simulink model "StopwatchAndrea"  (R2018b)
settings: Solver=FixedStepAuto  StartTime=0.0  StopTime=Inf  FixedStep=0.1  RelTol=1e-3
libraries: simulink x1
settings Model: Creator=user  LastModifiedBy=Andrea Stevanato
settings DataIOCC: LimitDataPoints=on
settings OptimizationCC: DefaultParameterBehavior=Inlined  EnhancedBackFolding=on  PassReuseOutputArgsAs=Individual arguments  OptimizeBlockOrder=speed  DifferentSizesBufferReuse=on  OptimizationCustomize=off
settings DebuggingCC: ParameterTunabilityLossMsg=error  AllowSymbolicDim=off  SFUnexpectedBacktrackingDiag=warning  SFNoUnconditionalDefaultTransitionDiag=warning  SFExecutionAtInitializationDiag=none
settings ModelReferenceCC: PropagateSignalLabelsOutOfModel=off
settings SFSimCC: SimUseLocalCustomCode=off  MATLABDynamicMemAlloc=off
settings RTWCC: SystemTargetFile=ert.tlc  GenCodeOnly=on  TemplateMakefile=ert_default_tmf  GenerateReport=on  RTWUseLocalCustomCode=off  IncludeHyperlinkInReport=on  LaunchReport=on  GenerateTraceInfo=on  GenerateTraceReport=on  GenerateTraceReportSl=on  GenerateTraceReportSf=on  GenerateTraceReportEml=on
settings CodeAppCC: ForceParamTrailComments=on  IgnoreCustomStorageClasses=off  OperatorAnnotations=on  SimulinkDataObjDesc=on  SFDataObjDesc=on  InsertBlockDesc=on
settings ERTTargetCC: IncludeMdlTerminateFcn=off  SupportAbsoluteTime=off  MultiInstanceERTCode=on  CodeInterfacePackaging=Reusable function  PurelyIntegerCode=on  SupportNonFinite=off  SupportComplex=off  GenerateAllocFcn=on  InlinedParameterPlacement=NonHierarchical  ERTCustomFileTemplate=example_file_process.tlc
settings ConfigComp: CovMetricSettings=dw  CovHtmlReporting=on  CovSaveCumulativeToWorkspaceVar=on  CovSaveSingleToWorkspaceVar=on  CovExternalEMLEnable=off

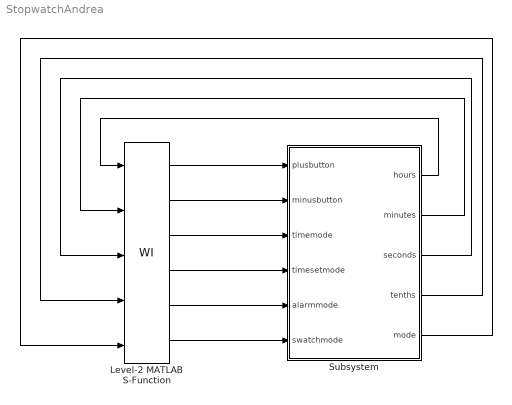
== system StopwatchAndrea ==
  Level-2 MATLAB S-Function : M-S-Function  FunctionName=WI
  Subsystem : Subsystem
  wires:
  Level-2 MATLAB S-Function/1 -> Subsystem/1(plusbutton)
  Level-2 MATLAB S-Function/2 -> Subsystem/2(minusbutton)
  Level-2 MATLAB S-Function/3 -> Subsystem/3(timemode)
  Level-2 MATLAB S-Function/4 -> Subsystem/4(timesetmode)
  Level-2 MATLAB S-Function/5 -> Subsystem/5(alarmmode)
  Level-2 MATLAB S-Function/6 -> Subsystem/6(swatchmode)
  Subsystem/1(hours) -> Level-2 MATLAB S-Function/1
  Subsystem/2(minutes) -> Level-2 MATLAB S-Function/2
  Subsystem/3(seconds) -> Level-2 MATLAB S-Function/3
  Subsystem/4(tenths) -> Level-2 MATLAB S-Function/4
  Subsystem/5(mode) -> Level-2 MATLAB S-Function/5

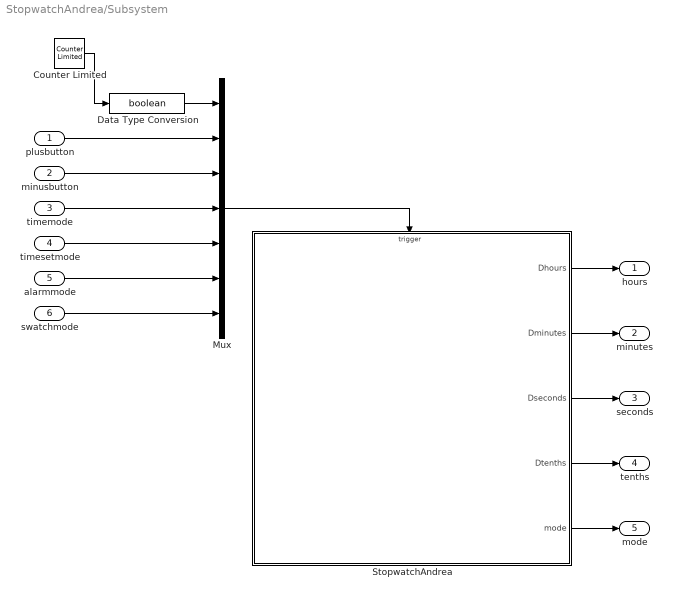
== system StopwatchAndrea/Subsystem ==
  plusbutton : Inport
  minusbutton : Inport  Port=2
  timemode : Inport  Port=3
  timesetmode : Inport  Port=4
  alarmmode : Inport  Port=5
  swatchmode : Inport  Port=6
  Counter Limited : simulink/Sources/Counter Limited  uplimit=1  tsamp=0.1
  Data Type Conversion : DataTypeConversion  OutDataTypeStr=boolean
  Mux : Mux  Inputs=7
  "StopwatchAndrea " : Stateflow chart  TreatAsAtomicUnit=on
  hours : Outport
  minutes : Outport  Port=2
  seconds : Outport  Port=3
  tenths : Outport  Port=4
  mode : Outport  Port=5
  wires:
  "StopwatchAndrea "/1(Dhours) -> hours/1
  Data Type Conversion/1 -> Mux/1
  Counter Limited/1 -> Data Type Conversion/1
  timemode/1 -> Mux/4
  timesetmode/1 -> Mux/5
  Mux/1 -> "StopwatchAndrea "/Trigger
  "StopwatchAndrea "/2(Dminutes) -> minutes/1
  "StopwatchAndrea "/3(Dseconds) -> seconds/1
  minusbutton/1 -> Mux/3
  "StopwatchAndrea "/5(mode) -> mode/1
  "StopwatchAndrea "/4(Dtenths) -> tenths/1
  alarmmode/1 -> Mux/6
  swatchmode/1 -> Mux/7
  plusbutton/1 -> Mux/2

== stateflow chart StopwatchAndrea/Subsystem/StopwatchAndrea  ==
  state Alarm [parallel]
    settings: executionOrder=2
    state Not_Setted
    state Silent
    state Buzzing
    Not_Setted -> Silent : [Ahours ~= 0 || Aminutes ~= 0]
    Silent -> Buzzing [order 1] : [Ahours==hours && Aminutes==minutes]
    (default) -> Not_Setted : {Ahours=uint8(0); Aminutes=uint8(0)}
    Silent -> Not_Setted [order 2] : [Ahours == 0 && Aminutes == 0]
    Buzzing -> Silent : Alarmmode[mode == 2]
  state Interface [parallel]
    settings: executionOrder=3
    state TimeDispaly
      en: mode=uint8(0)
      du: Dhours=hours; Dminutes=minutes; Dseconds=seconds; Dtenths=tenths;
    state TimeSet
      en: mode=uint8(1)
      state SetMinutes
        du: Dhours=hours; Dminutes=minutes
      state SetHours
        du: Dhours=hours; Dminutes=minutes
      SetMinutes -> SetMinutes [order 1] : plusbutton/{minutes=mod(minutes+1, 60)}
      SetHours -> SetHours [order 1] : plusbutton/{hours=mod(hours+1, 24)}
      SetHours -> SetMinutes [order 2] : Timesetmode
      (default) -> SetHours
      SetMinutes -> SetHours [order 2] : Timesetmode
      SetHours -> SetHours [order 3] : minusbutton/{hours=mod(hours+24-1,24)}
      SetMinutes -> SetMinutes [order 3] : minusbutton/{minutes=mod(minutes+60-1,60)}
    state Stopwatch
      en: mode=uint8(3)
      state Display
        du: Dhours=Shours; Dminutes=Sminutes; Dseconds=Sseconds; Dtenths=Stenths;
      state Partial
        en: Dhours=Phours; Dminutes=Pminutes; Dseconds=Pseconds; Dtenths=Ptenths;
      Stopwatch -> (history) [order 1] : Swatchmode
      (default) -> Display
      Display -> Partial : minusbutton{Phours=Shours; Pminutes=Sminutes; Pseconds=Sseconds; Ptenths=Stenths}
      Partial -> Display : minusbutton
    state AlarmSet
      en: mode=uint8(2)
      state SetHours1
        du: Dhours=Ahours; Dminutes=Aminutes
      state SetMinutes1
        du: Dhours=Ahours; Dminutes=Aminutes
      SetHours1 -> SetHours1 [order 1] : plusbutton/{Ahours=mod(Ahours+1, 24)}
      SetMinutes1 -> SetMinutes1 [order 1] : plusbutton/{Aminutes=mod(Aminutes+1, 60)}
      SetHours1 -> SetMinutes1 [order 3] : Alarmmode
      (default) -> SetHours1
      SetMinutes1 -> SetHours1 [order 3] : Alarmmode
      SetMinutes1 -> SetMinutes1 [order 2] : minusbutton/{Aminutes=mod(Aminutes+60-1, 60)}
      SetHours1 -> SetHours1 [order 2] : minusbutton/{Ahours=mod(Ahours+24-1, 24)}
    Interface -> TimeDispaly : Timemode
    (default) -> TimeDispaly : {Dhours=uint8(0); Dminutes=uint8(0); Dseconds=uint8(0); Dtenths=uint8(0);}
    TimeDispaly -> Stopwatch [order 3] : Swatchmode
    TimeDispaly -> AlarmSet [order 2] : Alarmmode
    TimeDispaly -> TimeSet [order 1] : Timesetmode
    TimeSet -> Stopwatch [order 2] : Swatchmode
    Stopwatch -> TimeSet [order 1] : Timesetmode
    Stopwatch -> AlarmSet [order 2] : Alarmmode
    AlarmSet -> Stopwatch [order 2] : Swatchmode
    AlarmSet -> TimeSet [order 1] : Timesetmode
    TimeSet -> AlarmSet [order 1] : Alarmmode
  state Timecount [parallel]
    settings: executionOrder=1
    state StopwatchCount [parallel]
      settings: executionOrder=1
      state Counting
      state NotCounting
      (junction 150) -> Counting [order 2] : /{Stenths=Stenths+1}
      (default) -> NotCounting : {Stenths = uint8(0); Sseconds = uint8(0); Sminutes = uint8(0); Shours = uint8(0)}
      (junction 150) -> (junction 148) [order 1] : [Stenths==9]/{Stenths=uint8(0)}
      (junction 148) -> (junction 156) [order 1] : [Sseconds==59]/{Sseconds=uint8(0)}
      NotCounting -> Counting [order 1] : plusbutton[mode==3]
      Counting -> (junction 150) [order 1] : Tick
      (junction 156) -> (junction 153) [order 1] : [Sminutes==59]/{Sminutes=uint8(0)}
      (junction 148) -> Counting [order 2] : /{Sseconds=Sseconds+1}
      (junction 156) -> Counting [order 2] : /{Sminutes=Sminutes+1}
      Counting -> NotCounting [order 2] : plusbutton[mode==3]
      NotCounting -> NotCounting [order 2] : Swatchmode[mode==3]/
          | {Stenths = uint8(0); Sseconds = uint8(0); Sminutes = uint8(0); Shours = uint8(0)}
      (junction 153) -> Counting : /{Shours=mod(Shours+1, 24)}
    state ClockCount [parallel]
      settings: executionOrder=2
      state Count
      (junction 108) -> Count [order 2] : /{tenths=tenths+1}
      (junction 108) -> (junction 109) [order 1] : [tenths==9]/{tenths=uint8(0)}
      (junction 109) -> (junction 110) [order 1] : [seconds==59]/{seconds=uint8(0)}
      Count -> (junction 108) : Tick
      (junction 110) -> (junction 114) [order 1] : [minutes==59]/{minutes=uint8(0)}
      (default) -> Count : {hours=uint8(0); minutes=uint8(0); seconds=uint8(0); tenths=uint8(0);}
      (junction 109) -> Count [order 2] : /{seconds=seconds+1}
      (junction 110) -> Count [order 2] : /{minutes=minutes+1}
      (junction 114) -> Count : /{hours=mod(hours+1, 24)}
  data: Dhours output uint8; Dminutes output uint8; Dseconds output uint8; Dtenths output uint8; mode output uint8; Ahours local uint8; Aminutes local uint8; hours local uint8; minutes local uint8; seconds local uint8; tenths local uint8; Shours local uint8; Sminutes local uint8; Sseconds local uint8; Stenths local uint8; Phours local uint8; Pminutes local uint8; Pseconds local uint8; Ptenths local uint8
  events: Tick input EITHER_EDGE_EVENT; plusbutton input RISING_EDGE_EVENT; minusbutton input RISING_EDGE_EVENT; Timemode input RISING_EDGE_EVENT; Timesetmode input RISING_EDGE_EVENT; Alarmmode input RISING_EDGE_EVENT; Swatchmode input RISING_EDGE_EVENT
